simulink model "magball_linear"  (R2023b)
settings: Solver=VariableStepAuto  StartTime=0.0  StopTime=2  RelTol=1e-3
undefined symbols (not defined in the file): i0, L, M, R, y0
settings Model: Creator=xiaom  LastModifiedBy=cr

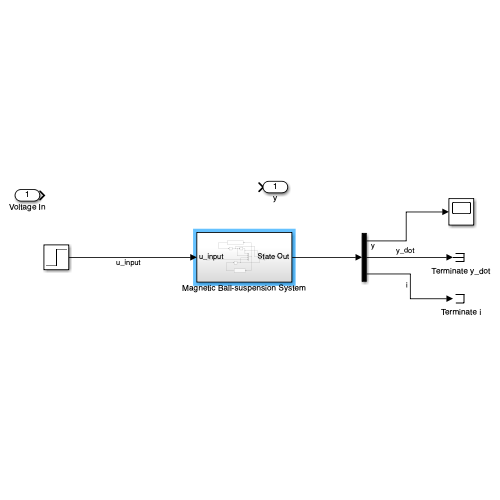
[thumbnail: Simulink's stored preview of the top-level diagram]
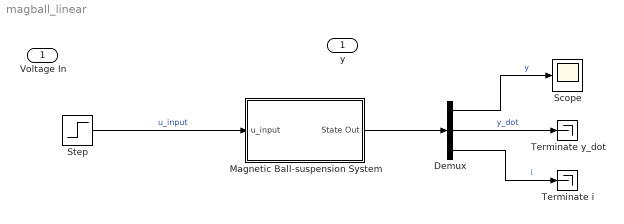
== system magball_linear ==
  Voltage In : Inport
  Demux : Demux  Outputs=3
  Magnetic Ball-suspension System : Subsystem
  Scope : Scope
  Step : Step  Time=0  SampleTime=0
  Terminate i : Terminator
  Terminate y_dot : Terminator
  y : Outport
  wires:
  Magnetic Ball-suspension System/1(State Out) -> Demux/1
  Demux/1 -> Scope/1  "y"
  Demux/3 -> Terminate i/1  "i"
  Demux/2 -> Terminate y_dot/1  "y_dot"
  Step/1 -> Magnetic Ball-suspension System/1(u_input)  "u_input"

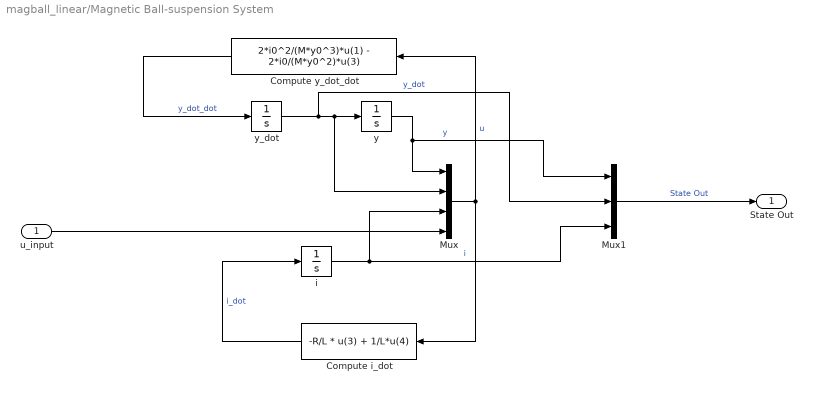
== system magball_linear/Magnetic Ball-suspension System ==
  u_input : Inport
  Compute i_dot : Fcn  Expr=-R/L * u(3) + 1/L*u(4)
  Compute y_dot_dot : Fcn  Expr=2*i0^2/(M*y0^3)*u(1) - 2*i0/(M*y0^2)*u(3)
  Mux : Mux
  Mux1 : Mux  Inputs=3
  i : Integrator
  y : Integrator
  y_dot : Integrator
  State Out : Outport
  wires:
  Mux1/1 -> State Out/1  "State Out"
  Compute i_dot/1 -> i/1  "i_dot"
  y_dot/1 -> Mux1/2, Mux/2, y/1  "y_dot"
  Mux/1 -> Compute i_dot/1, Compute y_dot_dot/1  "u"
  i/1 -> Mux1/3, Mux/3  "i"
  u_input/1 -> Mux/4
  Compute y_dot_dot/1 -> y_dot/1  "y_dot_dot"
  y/1 -> Mux1/1, Mux/1  "y"
